simulink model "TST_InjCrv_PiI2Set"  (R2016b)
settings: Solver=FixedStepDiscrete  StartTime=0.0  StopTime=simTime  FixedStep=sampleTime  RelTol=1e-3
values from neighbouring files (symbols this model uses):
  testCase = 1    [initTST_InjCrv_PiI2Set_001.m]
libraries: simulink x5, UnitTest_Lib x3
settings Model: Creator=zhengjinyan  LastModifiedBy=zhengjinyan
settings DebuggingCC: SignalRangeChecking=error

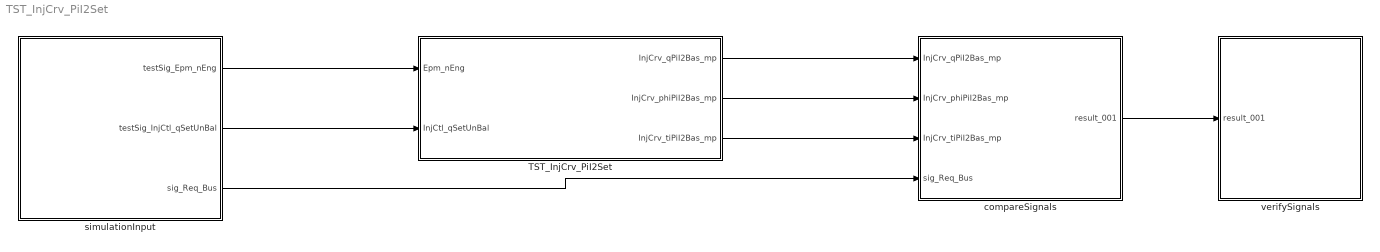
== system TST_InjCrv_PiI2Set ==
  TST_InjCrv_PiI2Set : Subsystem
  compareSignals : Subsystem
  simulationInput : Subsystem
  verifySignals : Subsystem
  wires:
  simulationInput/1(testSig_Epm_nEng) -> TST_InjCrv_PiI2Set/1(Epm_nEng)
  simulationInput/2(testSig_InjCtl_qSetUnBal) -> TST_InjCrv_PiI2Set/2(InjCtl_qSetUnBal)
  TST_InjCrv_PiI2Set/1(InjCrv_qPiI2Bas_mp) -> compareSignals/1(InjCrv_qPiI2Bas_mp)
  TST_InjCrv_PiI2Set/2(InjCrv_phiPiI2Bas_mp) -> compareSignals/2(InjCrv_phiPiI2Bas_mp)
  TST_InjCrv_PiI2Set/3(InjCrv_tiPiI2Bas_mp) -> compareSignals/3(InjCrv_tiPiI2Bas_mp)
  simulationInput/3(sig_Req_Bus) -> compareSignals/4(sig_Req_Bus)
  compareSignals/1(result_001) -> verifySignals/1(result_001)

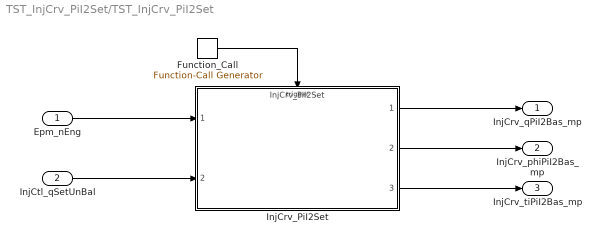
== system TST_InjCrv_PiI2Set/TST_InjCrv_PiI2Set ==
  Epm_nEng : Inport
  InjCtl_qSetUnBal : Inport  Port=2
  Function_Call : simulink/Ports & Subsystems/Function-Call Generator  sample_time=sampleTime  numberOfIterations=1
  InjCrv_PiI2Set : ModelReference  ModelNameDialog=InjCrv_PiI2Set  SimulationMode=Normal  ModelReferenceVersion=1.17  TriggerPortName=function  TriggerPortTriggerType=function-call  TriggerPortStatesWhenEnabling=held
  InjCrv_qPiI2Bas_mp : Outport
  InjCrv_phiPiI2Bas_mp : Outport  Port=2
  InjCrv_tiPiI2Bas_mp : Outport  Port=3
  wires:
  Function_Call/1 -> InjCrv_PiI2Set/Trigger
  Epm_nEng/1 -> InjCrv_PiI2Set/1
  InjCtl_qSetUnBal/1 -> InjCrv_PiI2Set/2
  InjCrv_PiI2Set/1 -> InjCrv_qPiI2Bas_mp/1
  InjCrv_PiI2Set/2 -> InjCrv_phiPiI2Bas_mp/1
  InjCrv_PiI2Set/3 -> InjCrv_tiPiI2Bas_mp/1

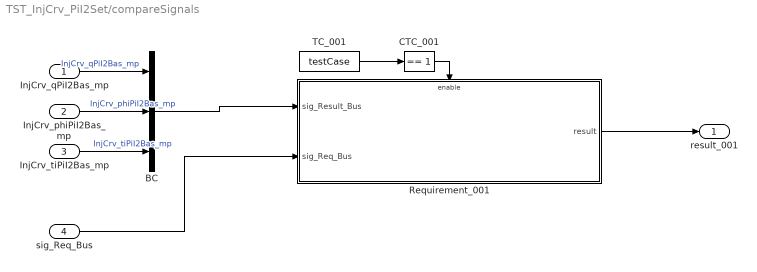
== system TST_InjCrv_PiI2Set/compareSignals ==
  InjCrv_qPiI2Bas_mp : Inport
  InjCrv_phiPiI2Bas_mp : Inport  Port=2
  InjCrv_tiPiI2Bas_mp : Inport  Port=3
  sig_Req_Bus : Inport  Port=4
  BC : BusCreator  Inputs=3
  CTC_001 : simulink/Logic and Bit Operations/Compare To Constant  relop===  const=1  OutDataTypeStr=boolean
  Requirement_001 : Subsystem
  TC_001 : Constant  Value=testCase
  result_001 : Outport
  wires:
  InjCrv_qPiI2Bas_mp/1 -> BC/1  "InjCrv_qPiI2Bas_mp"
  InjCrv_phiPiI2Bas_mp/1 -> BC/2  "InjCrv_phiPiI2Bas_mp"
  InjCrv_tiPiI2Bas_mp/1 -> BC/3  "InjCrv_tiPiI2Bas_mp"
  TC_001/1 -> CTC_001/1
  CTC_001/1 -> Requirement_001/Enable
  sig_Req_Bus/1 -> Requirement_001/2(sig_Req_Bus)
  BC/1 -> Requirement_001/1(sig_Result_Bus)
  Requirement_001/1(result) -> result_001/1

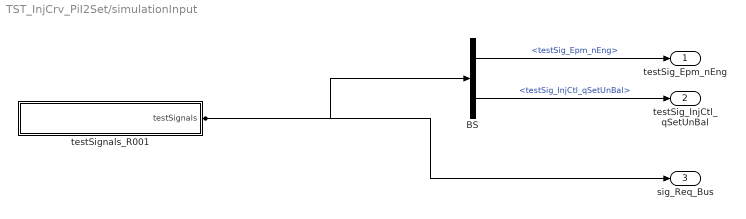
== system TST_InjCrv_PiI2Set/simulationInput ==
  BS : BusSelector  OutputSignals=testSig_Epm_nEng,testSig_InjCtl_qSetUnBal
  testSignals_R001 : Subsystem
  testSig_Epm_nEng : Outport
  testSig_InjCtl_qSetUnBal : Outport  Port=2
  sig_Req_Bus : Outport  Port=3
  wires:
  BS/1 -> testSig_Epm_nEng/1  "<testSig_Epm_nEng>"
  BS/2 -> testSig_InjCtl_qSetUnBal/1  "<testSig_InjCtl_qSetUnBal>"
  testSignals_R001/1(testSignals) -> BS/1, sig_Req_Bus/1

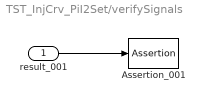
== system TST_InjCrv_PiI2Set/verifySignals ==
  result_001 : Inport
  Assertion_001 : Assertion  Enabled=off
  wires:
  result_001/1 -> Assertion_001/1

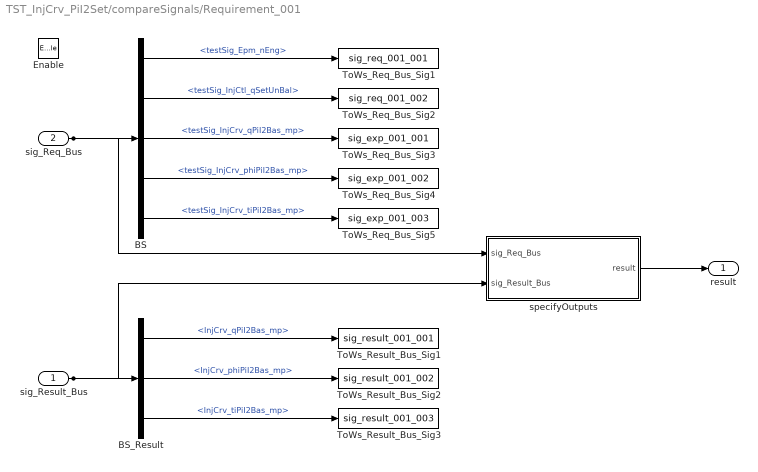
== system TST_InjCrv_PiI2Set/compareSignals/Requirement_001 ==
  sig_Result_Bus : Inport
  sig_Req_Bus : Inport  Port=2
  Enable : EnablePort
  BS : BusSelector  OutputSignals=testSig_Epm_nEng,testSig_InjCtl_qSetUnBal,testSig_InjCrv_qPiI2Bas_mp,testSig_InjCrv_phiPiI2Bas_mp,testSig_InjCrv_tiPiI2Bas_mp
  BS_Result : BusSelector  OutputSignals=InjCrv_qPiI2Bas_mp,InjCrv_phiPiI2Bas_mp,InjCrv_tiPiI2Bas_mp
  ToWs_Req_Bus_Sig1 : ToWorkspace  VariableName=sig_req_001_001  SaveFormat=Structure With Time
  ToWs_Req_Bus_Sig2 : ToWorkspace  VariableName=sig_req_001_002  SaveFormat=Structure With Time
  ToWs_Req_Bus_Sig3 : ToWorkspace  VariableName=sig_exp_001_001  SaveFormat=Structure With Time
  ToWs_Req_Bus_Sig4 : ToWorkspace  VariableName=sig_exp_001_002  SaveFormat=Structure With Time
  ToWs_Req_Bus_Sig5 : ToWorkspace  VariableName=sig_exp_001_003  SaveFormat=Structure With Time
  ToWs_Result_Bus_Sig1 : ToWorkspace  VariableName=sig_result_001_001  SaveFormat=Structure With Time
  ToWs_Result_Bus_Sig2 : ToWorkspace  VariableName=sig_result_001_002  SaveFormat=Structure With Time
  ToWs_Result_Bus_Sig3 : ToWorkspace  VariableName=sig_result_001_003  SaveFormat=Structure With Time
  specifyOutputs : Subsystem
  result : Outport
  wires:
  sig_Req_Bus/1 -> BS/1, specifyOutputs/1(sig_Req_Bus)
  BS/1 -> ToWs_Req_Bus_Sig1/1  "<testSig_Epm_nEng>"
  BS/2 -> ToWs_Req_Bus_Sig2/1  "<testSig_InjCtl_qSetUnBal>"
  BS/3 -> ToWs_Req_Bus_Sig3/1  "<testSig_InjCrv_qPiI2Bas_mp>"
  BS/4 -> ToWs_Req_Bus_Sig4/1  "<testSig_InjCrv_phiPiI2Bas_mp>"
  BS/5 -> ToWs_Req_Bus_Sig5/1  "<testSig_InjCrv_tiPiI2Bas_mp>"
  sig_Result_Bus/1 -> BS_Result/1, specifyOutputs/2(sig_Result_Bus)
  BS_Result/1 -> ToWs_Result_Bus_Sig1/1  "<InjCrv_qPiI2Bas_mp>"
  BS_Result/2 -> ToWs_Result_Bus_Sig2/1  "<InjCrv_phiPiI2Bas_mp>"
  BS_Result/3 -> ToWs_Result_Bus_Sig3/1  "<InjCrv_tiPiI2Bas_mp>"
  specifyOutputs/1(result) -> result/1

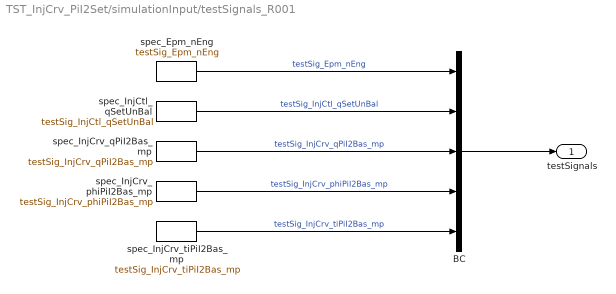
== system TST_InjCrv_PiI2Set/simulationInput/testSignals_R001 ==
  BC : BusCreator  Inputs=5
  spec_Epm_nEng : FromWorkspace  VariableName=testSig_Epm_nEng  Interpolate=off  OutputAfterFinalValue=Holding final value
  spec_InjCrv_phiPiI2Bas_mp : FromWorkspace  VariableName=testSig_InjCrv_phiPiI2Bas_mp  Interpolate=off  OutputAfterFinalValue=Holding final value
  spec_InjCrv_qPiI2Bas_mp : FromWorkspace  VariableName=testSig_InjCrv_qPiI2Bas_mp  Interpolate=off  OutputAfterFinalValue=Holding final value
  spec_InjCrv_tiPiI2Bas_mp : FromWorkspace  VariableName=testSig_InjCrv_tiPiI2Bas_mp  Interpolate=off  OutputAfterFinalValue=Holding final value
  spec_InjCtl_qSetUnBal : FromWorkspace  VariableName=testSig_InjCtl_qSetUnBal  Interpolate=off  OutputAfterFinalValue=Holding final value
  testSignals : Outport
  wires:
  BC/1 -> testSignals/1
  spec_Epm_nEng/1 -> BC/1  "testSig_Epm_nEng"
  spec_InjCtl_qSetUnBal/1 -> BC/2  "testSig_InjCtl_qSetUnBal"
  spec_InjCrv_qPiI2Bas_mp/1 -> BC/3  "testSig_InjCrv_qPiI2Bas_mp"
  spec_InjCrv_phiPiI2Bas_mp/1 -> BC/4  "testSig_InjCrv_phiPiI2Bas_mp"
  spec_InjCrv_tiPiI2Bas_mp/1 -> BC/5  "testSig_InjCrv_tiPiI2Bas_mp"

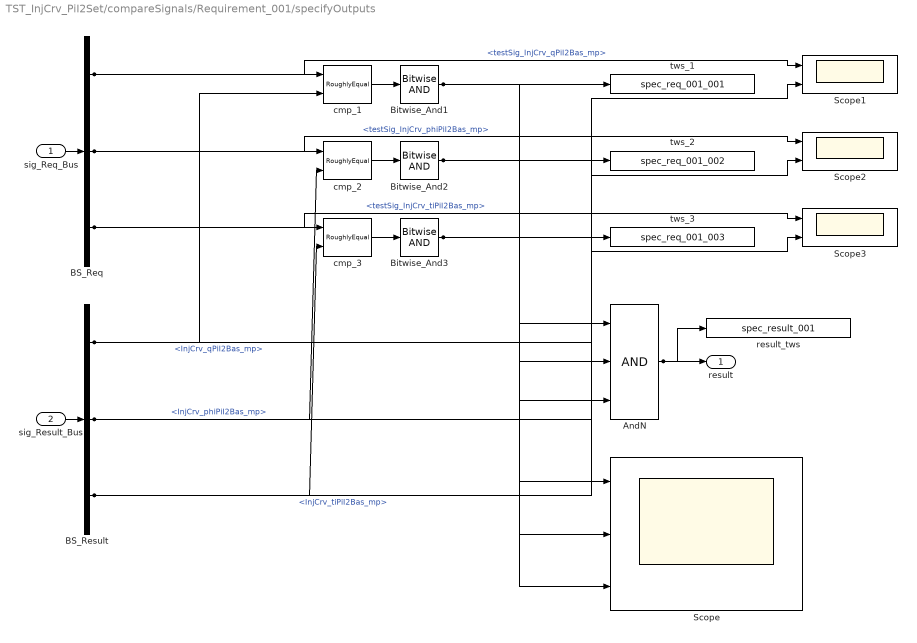
== system TST_InjCrv_PiI2Set/compareSignals/Requirement_001/specifyOutputs ==
  sig_Req_Bus : Inport
  sig_Result_Bus : Inport  Port=2
  AndN : Logic  Inputs=3
  BS_Req : BusSelector  OutputSignals=testSig_InjCrv_qPiI2Bas_mp,testSig_InjCrv_phiPiI2Bas_mp,testSig_InjCrv_tiPiI2Bas_mp
  BS_Result : BusSelector  OutputSignals=InjCrv_qPiI2Bas_mp,InjCrv_phiPiI2Bas_mp,InjCrv_tiPiI2Bas_mp
  Bitwise_And1 : simulink/Logic and Bit Operations/Bitwise Operator  logicop=AND  UseBitMask=off  BitMask=bin2dec('11011001')  BitMaskRealWorld=Stored Integer
  Bitwise_And2 : simulink/Logic and Bit Operations/Bitwise Operator  logicop=AND  UseBitMask=off  BitMask=bin2dec('11011001')  BitMaskRealWorld=Stored Integer
  Bitwise_And3 : simulink/Logic and Bit Operations/Bitwise Operator  logicop=AND  UseBitMask=off  BitMask=bin2dec('11011001')  BitMaskRealWorld=Stored Integer
  Scope : Scope  NumInputPorts=3
  Scope1 : Scope  NumInputPorts=2
  Scope2 : Scope  NumInputPorts=2
  Scope3 : Scope  NumInputPorts=2
  cmp_1 : UnitTest_Lib/RoughlyEqual  slope=0.1
  cmp_2 : UnitTest_Lib/RoughlyEqual  slope=0.1
  cmp_3 : UnitTest_Lib/RoughlyEqual  slope=0.1
  result_tws : ToWorkspace  VariableName=spec_result_001
  tws_1 : ToWorkspace  VariableName=spec_req_001_001
  tws_2 : ToWorkspace  VariableName=spec_req_001_002
  tws_3 : ToWorkspace  VariableName=spec_req_001_003
  result : Outport
  wires:
  sig_Req_Bus/1 -> BS_Req/1
  sig_Result_Bus/1 -> BS_Result/1
  AndN/1 -> result/1, result_tws/1
  BS_Req/1 -> cmp_1/1, Scope1/1  "<testSig_InjCrv_qPiI2Bas_mp>"
  BS_Result/1 -> cmp_1/2, Scope1/2  "<InjCrv_qPiI2Bas_mp>"
  cmp_1/1 -> Bitwise_And1/1
  Bitwise_And1/1 -> tws_1/1, AndN/1, Scope/1
  BS_Req/2 -> cmp_2/1, Scope2/1  "<testSig_InjCrv_phiPiI2Bas_mp>"
  BS_Result/2 -> cmp_2/2, Scope2/2  "<InjCrv_phiPiI2Bas_mp>"
  cmp_2/1 -> Bitwise_And2/1
  Bitwise_And2/1 -> tws_2/1, AndN/2, Scope/2
  BS_Req/3 -> cmp_3/1, Scope3/1  "<testSig_InjCrv_tiPiI2Bas_mp>"
  BS_Result/3 -> cmp_3/2, Scope3/2  "<InjCrv_tiPiI2Bas_mp>"
  cmp_3/1 -> Bitwise_And3/1
  Bitwise_And3/1 -> tws_3/1, AndN/3, Scope/3
